simulink model "reduced_order_observer_controller_simulation"  (R2016a)
settings: Solver=VariableStepAuto  StartTime=0.0  StopTime=20.0  RelTol=1e-3
values from neighbouring files (symbols this model uses):
  a = obj.a    [System.m]    (also in system_examples.m = [-15,-14,-24;-14,-14,-24;15,15,25])
  b = obj.b    [System.m]    (also in system_examples.m = [1;1;-1])
  c = obj.c    [System.m]    (also in system_examples.m = [1,1,2])
  css = eye(size(a))    [System.m]
  dss = [zeros(size(a,1), 1)]    [System.m]
  k = place(an, bn, des_eigs)    [System.m]    (also in system_examples.m = ol_sys.get_control_gain(des_poles))
  l = obj.full_observer_gain(des_eigs)    [System.m]
  x0 = obj.x0    [System.m]
undefined symbols (not defined in the file or in its folder): ap, aq, e_m_lc, pt, qt
settings Model: Creator=micah  LastModifiedBy=micah

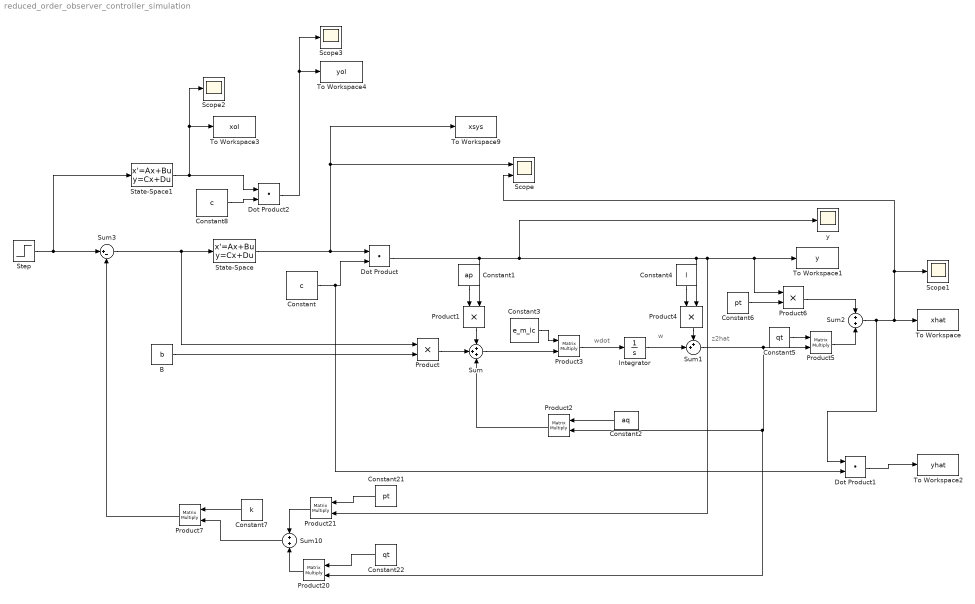
== system reduced_order_observer_controller_simulation ==
  note: z2hat
  note: w
  note: wdot
  B : Constant  Value=b  VectorParams1D=off
  Constant : Constant  Value=c
  Constant1 : Constant  Value=ap
  Constant2 : Constant  Value=aq
  Constant21 : Constant  Value=pt  VectorParams1D=off
  Constant22 : Constant  Value=qt  VectorParams1D=off
  Constant3 : Constant  Value=e_m_lc
  Constant4 : Constant  Value=l
  Constant5 : Constant  Value=qt
  Constant6 : Constant  Value=pt
  Constant7 : Constant  Value=k  VectorParams1D=off
  Constant8 : Constant  Value=c
  Dot Product : DotProduct  InputSameDT=on  OutDataTypeStr=Inherit: Inherit via internal rule
  Dot Product1 : DotProduct  InputSameDT=on  OutDataTypeStr=Inherit: Inherit via internal rule
  Dot Product2 : DotProduct  InputSameDT=on  OutDataTypeStr=Inherit: Inherit via internal rule
  Integrator : Integrator
  Product{,1,4,6} (4 alike) : Product
  Product{2..3,5,7,20..21} (6 alike) : Product  Multiplication=Matrix(*)
  Scope : Scope  NumInputPorts=2
  Scope1 : Scope
  Scope2 : Scope
  Scope3 : Scope
  State-Space : StateSpace  A=a  B=b  C=css  D=dss  X0=x0
  State-Space1 : StateSpace  A=a  B=b  C=css  D=dss  X0=x0
  Step : Step  Time=0  SampleTime=0
  Sum : Sum  Inputs=+++
  Sum1 : Sum  Inputs=++|
  Sum10 : Sum  Inputs=+|+
  Sum2 : Sum  Inputs=+|+
  Sum3 : Sum  Inputs=|+-
  To Workspace : ToWorkspace  VariableName=xhat  SaveFormat=Structure With Time  SampleTime=-1
  To Workspace1 : ToWorkspace  VariableName=y  SaveFormat=Structure With Time  SampleTime=-1
  To Workspace2 : ToWorkspace  VariableName=yhat  SaveFormat=Structure With Time  SampleTime=-1
  To Workspace3 : ToWorkspace  VariableName=xol  SaveFormat=Structure With Time  SampleTime=-1
  To Workspace4 : ToWorkspace  VariableName=yol  SaveFormat=Structure With Time  SampleTime=-1
  To Workspace9 : ToWorkspace  VariableName=xsys  SaveFormat=Structure With Time  SampleTime=-1
  y : Scope
  wires:
  Sum3/1 -> Product/1, State-Space/1
  State-Space/1 -> To Workspace9/1, Scope/1, Dot Product/1
  Constant/1 -> Dot Product1/2, Dot Product/2
  Dot Product/1 -> y/1, Product21/2, To Workspace1/1, Product6/1, Product4/2, Product1/2
  B/1 -> Product/2
  Product/1 -> Sum/2
  Constant1/1 -> Product1/1
  Product1/1 -> Sum/1
  Constant2/1 -> Product2/1
  Product2/1 -> Sum/3
  Sum/1 -> Product3/2
  Constant3/1 -> Product3/1
  Product3/1 -> Integrator/1
  Integrator/1 -> Sum1/2
  Constant4/1 -> Product4/1
  Product4/1 -> Sum1/1
  Sum1/1 -> Product5/2, Product20/2, Product2/2
  Constant5/1 -> Product5/1
  Constant6/1 -> Product6/2
  Product6/1 -> Sum2/1
  Product5/1 -> Sum2/2
  Sum2/1 -> Dot Product1/1, Scope1/1, Scope/2, To Workspace/1
  Dot Product1/1 -> To Workspace2/1
  Step/1 -> State-Space1/1, Sum3/1
  Constant7/1 -> Product7/1
  Product7/1 -> Sum3/2
  Sum10/1 -> Product7/2
  State-Space1/1 -> Scope2/1, To Workspace3/1, Dot Product2/1
  Constant8/1 -> Dot Product2/2
  Dot Product2/1 -> Scope3/1, To Workspace4/1
  Constant21/1 -> Product21/1
  Constant22/1 -> Product20/1
  Product20/1 -> Sum10/2
  Product21/1 -> Sum10/1
